simulink model "Train_with_data_R2021a"  (R2021a)
settings: Solver=FixedStepAuto  StartTime=0.0  StopTime=30  FixedStep=1/1000  RelTol=1e-3  EnableMultiTasking=on
libraries: rllib x1
settings Model: Creator=Ammar  LastModifiedBy=vic-b
settings SolverCC: AlgebraicLoopSolver=TrustRegion  PositivePriorityOrder=on  AutoInsertRateTranBlk=on
settings OptimizationCC: EnhancedBackFolding=on  PassReuseOutputArgsThreshold=0  MaxStackSize=64  OptimizeBlockOrder=speed  DifferentSizesBufferReuse=on  OptimizationCustomize=off
settings DebuggingCC: ParameterTunabilityLossMsg=error  SFMachineParentedDataDiag=warning  ArithmeticOperatorsInVariantConditions=warning
settings HardwareCC: ProdBitPerPointer=32  ProdBitPerSizeT=32  ProdBitPerPtrDiffT=32  ProdLargestAtomicInteger=Long  ProdLargestAtomicFloat=Double  ProdWordSize=32  ProdHWDeviceType=ARM Compatible->ARM Cortex  UseEmbeddedCoderFeatures=off  UseSimulinkCoderFeatures=off
settings SFSimCC: SimUseLocalCustomCode=off  MATLABDynamicMemAlloc=off  CustomCodeUndefinedFunction=UseInterfaceOnly  SimTargetLang=C++
settings RTWCC: SystemTargetFile=ert.tlc  HardwareBoard=Raspberry Pi  TLCOptions="-aInlineSetEventsForThisBaseRateFcn=TLC_FALSE -aSuppressMultiTaskScheduler=TLC_FALSE  -aRateBasedStepFcn=0"  TemplateMakefile=ert_default_tmf  GenerateReport=on  RTWUseLocalCustomCode=off  Toolchain=GNU GCC Embedded Linux  BuildConfiguration=Faster Runs  LaunchReport=on
settings CodeAppCC: ForceParamTrailComments=on  OperatorAnnotations=on
settings ERTTargetCC: ERTCustomFileBanners=off  SupportContinuousTime=on  SupportNonInlinedSFcns=on  RemoveResetFunc=off  SupportVariableSizeSignals=on  ModelStepFunctionPrototypeControlCompliant=off

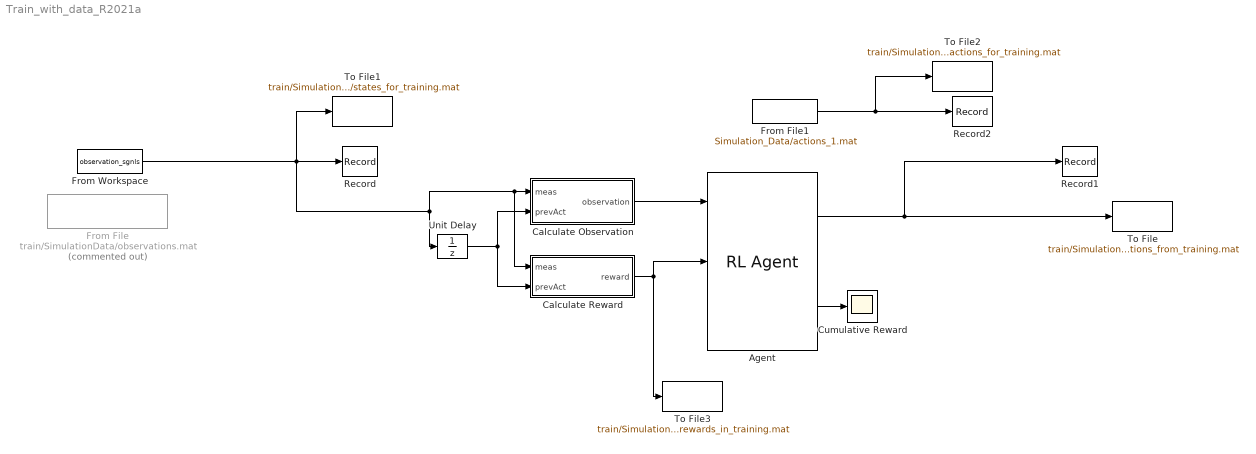
== system Train_with_data_R2021a ==
  Agent : rllib/RL Agent  Agent=agent  ExternalActionAsInput=off  ProvideCumRwd=on  TreatAsDirectFeedthrough=on
      settings: SourceProductName=Reinforcement Learning
  Calculate Observation : Subsystem
  Calculate Reward : Subsystem
  Cumulative Reward : Scope
  From Workspace : FromWorkspace  VariableName=observation_sgnls
  From File : FromFile  Commented=on  FileName=train/SimulationData/observations.mat  SampleTime=0.004
  From File1 : FromFile  FileName=Simulation_Data/actions_1.mat  SampleTime=0
  Record : Record  FileSettingsInternal="{\"entries\":[{\"content\":{\"excelSettings\":{\"content\":{},\"type\":\"Streamout.ExcelSettings\"}},\"type\":\"Streamout.FileSettingStorage\",\"uuid\":\"ed9f7456-e5c5-4088-b545-380a04e12139\"}],\"packageUris\":[\"http://schema.mathworks.com/mf0/streamout_blocks/R2020a\"],\"version\":\"1.0\"}"  Layout=[1 1]  SignalsInternal="{\"entries\":[{\"content\":{\"signals\":[{\"content\":{\"blockPath\":[\"Train_with_data_R2021a/Record\"],\"channel\":[],\"dimensions\":[1],\"domain\":\"train_with_data_r2021a/record\",\"lineColor\":\"#edb120\",\"plots\":[],\"port\":1,\"sid\":[\"\"],\"signalID\":1818,\"signalName\":\"From\\nWorkspace\"},\"type\":\"RecordBlkView.Signal\",\"uuid\":\"9fea5119-e826-46e6-bc0e-0e3670b1dc2c\"}]},\"type\":\"RecordBlkView.InputSignals\",\"uuid\":\"876ae538-406f-4c0d-9890-31d20bc8f578\"}],\"packageUris\":[\"http://schema.mathworks.com/mf0/streamout_blocks/R2020a\"],\"version\":\"1.0\"}"  VisualizationBindings="{\"sparklinesplugin\":{\"info\":[{\"bindingParametersList\":[],\"subplotID\":1}]}}"
  Record1 : Record  FileSettingsInternal="{\"entries\":[{\"content\":{\"excelSettings\":{\"content\":{},\"type\":\"Streamout.ExcelSettings\"}},\"type\":\"Streamout.FileSettingStorage\",\"uuid\":\"151a962a-1665-4290-9066-655ba5bfd431\"}],\"packageUris\":[\"http://schema.mathworks.com/mf0/streamout_blocks/R2020a\"],\"version\":\"1.0\"}"  SignalsInternal="{\"entries\":[{\"content\":{\"signals\":[{\"content\":{\"blockPath\":[\"Train_with_data_R2021a/Record1\"],\"channel\":[],\"dimensions\":[1,1],\"domain\":\"train_with_data_r2021a/record1\",\"lineColor\":\"#0072bd\",\"plots\":[1],\"port\":1,\"sid\":[\"\"],\"signalID\":1826,\"signalName\":\"Agent:1\"},\"type\":\"RecordBlkView.Signal\",\"uuid\":\"2af4a1d3-5544-4295-be56-dd9efd24aec9\"}]},\"type\":\"RecordBlkView.InputSignals\",\"uuid\":\"c4f9a41c-1898-48b3-9228-5177bd999cc0\"}],\"packageUris\":[\"http://schema.mathworks.com/mf0/streamout_blocks/R2020a\"],\"version\":\"1.0\"}"  VisualizationBindings="{\"sparklinesplugin\":{\"info\":[{\"bindingParametersList\":[],\"subplotID\":1}]}}"
  Record2 : Record  FileSettingsInternal="{\"entries\":[{\"content\":{\"excelSettings\":{\"content\":{},\"type\":\"Streamout.ExcelSettings\"}},\"type\":\"Streamout.FileSettingStorage\",\"uuid\":\"6a1205b6-9820-4cbd-98b7-17465b8ef8e2\"}],\"packageUris\":[\"http://schema.mathworks.com/mf0/streamout_blocks/R2020a\"],\"version\":\"1.0\"}"  SignalsInternal="{\"entries\":[{\"content\":{\"signals\":[{\"content\":{\"blockPath\":[\"Train_with_data_R2021a/Record2\"],\"channel\":[],\"dimensions\":[1,1],\"domain\":\"train_with_data_r2021a/record2\",\"lineColor\":\"#d95319\",\"plots\":[1],\"port\":1,\"sid\":[\"\"],\"signalID\":1822,\"signalName\":\"From File1\"},\"type\":\"RecordBlkView.Signal\",\"uuid\":\"a0e8b514-49e5-455b-9608-c86686f98b3f\"}]},\"type\":\"RecordBlkView.InputSignals\",\"uuid\":\"2de236d8-8c49-480b-abe2-db39c8c6ecaf\"}],\"packageUris\":[\"http://schema.mathworks.com/mf0/streamout_blocks/R2020a\"],\"version\":\"1.0\"}"  VisualizationBindings="{\"sparklinesplugin\":{\"info\":[{\"bindingParametersList\":[],\"subplotID\":1}]}}"
  To File : ToFile  Filename=train/SimulationData/actions_from_training.mat  SaveFormat=Timeseries
  To File1 : ToFile  Filename=train/SimulationData/states_for_training.mat  SaveFormat=Timeseries
  To File2 : ToFile  Filename=train/SimulationData/actions_for_training.mat  SaveFormat=Timeseries
  To File3 : ToFile  Filename=train/SimulationData/rewards_in_training.mat  SaveFormat=Timeseries
  Unit Delay : UnitDelay  SampleTime=-1  HasFrameUpgradeWarning=on
  wires:
  Calculate Observation/1(observation) -> Agent/1
  Unit Delay/1 -> Calculate Observation/2(prevAct), Calculate Reward/2(prevAct)
  Agent/2 -> Cumulative Reward/1
  Agent/1 -> To File/1, Record1/1
  Calculate Reward/1(reward) -> Agent/2, To File3/1
  From File1/1 -> To File2/1, Record2/1
  From Workspace/1 -> Calculate Reward/1(meas), Calculate Observation/1(meas), Unit Delay/1, Record/1, To File1/1

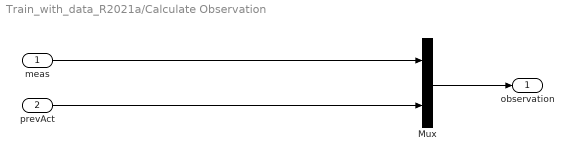
== system Train_with_data_R2021a/Calculate Observation ==
  meas : Inport
  prevAct : Inport  Port=2
  Mux : Mux  Inputs=2
  observation : Outport  VectorParamsAs1DForOutWhenUnconnected=off
  wires:
  Mux/1 -> observation/1
  meas/1 -> Mux/1
  prevAct/1 -> Mux/2

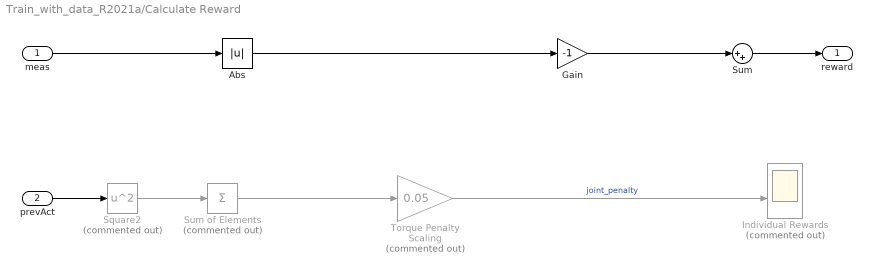
== system Train_with_data_R2021a/Calculate Reward ==
  meas : Inport
  prevAct : Inport  Port=2
  Abs : Abs
  Gain : Gain  Gain=-1
  Individual Rewards : Scope  Commented=on  NumInputPorts=4
  Square2 : Math  Commented=on  Operator=square  SignedPower=on  SaturateOnIntegerOverflow=on
  Sum : Sum  Inputs=|++
  Sum of Elements : Sum  Commented=on  Inputs=+
  Torque Penalty Scaling : Gain  Commented=on  Gain=0.05
  reward : Outport  VectorParamsAs1DForOutWhenUnconnected=off
  wires:
  meas/1 -> Abs/1
  Sum of Elements/1 -> Torque Penalty Scaling/1
  prevAct/1 -> Square2/1
  Square2/1 -> Sum of Elements/1
  Torque Penalty Scaling/1 -> Individual Rewards/3  "joint_penalty"
  Abs/1 -> Gain/1
  Gain/1 -> Sum/1
  Sum/1 -> reward/1
